simulink model "Multsines"  (R2015a)
settings: Solver=ode45  StartTime=0.0  StopTime=10.0  RelTol=1e-3
settings Model: Creator=Yuri  LastModifiedBy=Yuri

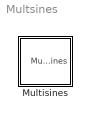
== system Multsines ==
  Multisines : Subsystem

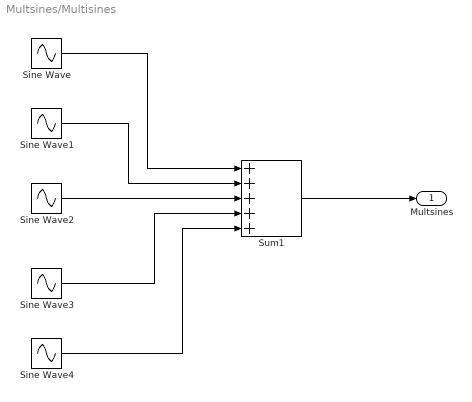
== system Multsines/Multisines ==
  Sine Wave : Sin  SampleTime=0
  Sine Wave1 : Sin  Frequency=1.9  Phase=-2*(2-1)*pi/5  SampleTime=0
  Sine Wave2 : Sin  Frequency=2.1  Phase=-3*(3-1)*pi/5  SampleTime=0
  Sine Wave3 : Sin  Frequency=22  Phase=-4*(4-1)*pi/5  SampleTime=0
  Sine Wave4 : Sin  Frequency=18  Phase=-5*(5-1)*pi/5  SampleTime=0
  Sum1 : Sum  Inputs=+++++
  "Multsines " : Outport
  wires:
  Sine Wave3/1 -> Sum1/4
  Sine Wave4/1 -> Sum1/5
  Sine Wave/1 -> Sum1/1
  Sine Wave2/1 -> Sum1/3
  Sine Wave1/1 -> Sum1/2
  Sum1/1 -> "Multsines "/1
